simulink model "sampleModel1903"  (R2023a)
settings: Solver=VariableStepAuto  StartTime=0.0  StopTime=10.0  RelTol=1e-3
libraries: hdlsllib x2, simulink x1
settings Model: Creator=user1  LastModifiedBy=user1

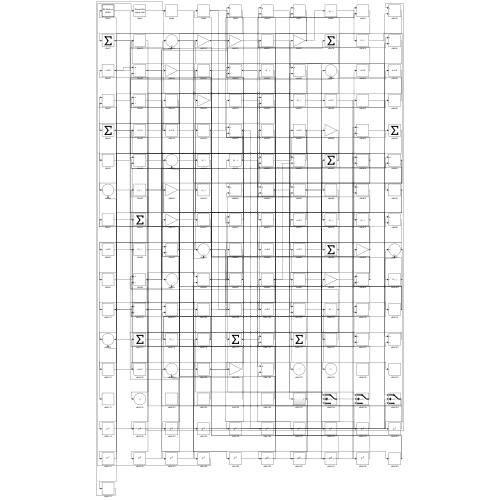
[thumbnail: Simulink's stored preview of the top-level diagram]
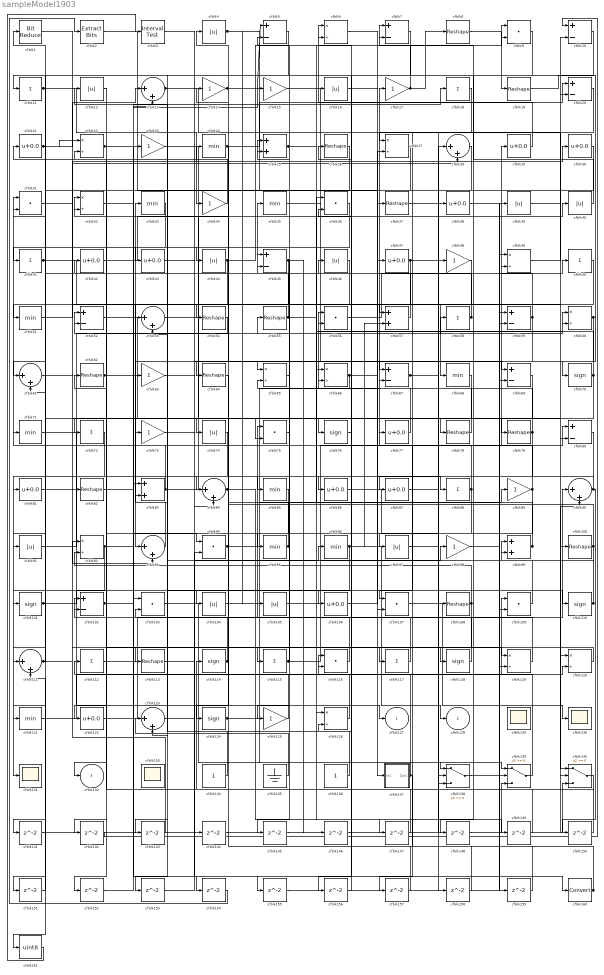
== system sampleModel1903 ==
  cfblk1 : hdlsllib/Logic and Bit Operations/Bit Reduce  mode=AND
  cfblk{5,7,10,20,45,52,59,67,69,80,102} (11 alike) : Sum  Inputs=+-
  cfblk{8,19,26,37,54..55,62,64,78..79,82,100,108,113} (14 alike) : Reshape
  cfblk{70,76,101,110,114,118,124} (7 alike) : Signum
  cfblk{9,31,36,56,75,94,103,107,109,116} (10 alike) : DotProduct  OutDataTypeStr=Inherit: Inherit via internal rule
  cfblk{4,12,16,39..40,44,46,74,91,97,104..105} (12 alike) : Abs  SaturateOnIntegerOverflow=off
  cfblk{21,29..30,38,42..43,47,77,81,86..87,106,122} (13 alike) : Bias  Bias=0.0  SaturateOnIntegerOverflow=off
  cfblk{11,18,41,50,58,72,88,112,115,117} (10 alike) : Sum  Inputs=+
  cfblk{13,28,53,61,84,90,93,111,123} (9 alike) : Sum  Inputs=|++
  cfblk{6,22,27,32,49,60,65..66,92,119..120,126} (12 alike) : Product  Inputs=*/  RndMeth=Zero  SaturateOnIntegerOverflow=on
  cfblk{24,33,35,51,68,71,85,95..96,121} (10 alike) : MinMax
  cfblk{14..15,17,23,34,48,63,73,89,98,125} (11 alike) : Gain
  cfblk{129..131,133} (4 alike) : Scope
      cfblk129 settings: Floating=on
      cfblk133 settings: Floating=on
  cfblk134 : Constant  SampleTime=-1
  cfblk135 : Ground
  cfblk136 : Constant  SampleTime=-1
  cfblk137 : Subsystem
      settings: LibrarySourceBlock=|
      | hdlsllib/Ports &
      | Subsystems/Subsystem
  cfblk138 : Switch  SaturateOnIntegerOverflow=off  InputSameDT=off
  cfblk139 : Switch  SaturateOnIntegerOverflow=off  InputSameDT=off
  cfblk140 : Switch  SaturateOnIntegerOverflow=off  InputSameDT=off
  cfblk{141..159} (19 alike) : Delay  SampleTime=1
  cfblk160 : DataTypeConversion  SaturateOnIntegerOverflow=off  RndMeth=Floor
  cfblk161 : DataTypeConversion  OutDataTypeStr=uint8  SaturateOnIntegerOverflow=off  RndMeth=Floor
  cfblk2 : simulink/Logic and Bit Operations/Extract Bits  bitsToExtract=Upper half  numBits=8  bitIdxRange=[0 7]  outScalingMode=Preserve fixed-point scaling
      settings: LibrarySourceBlock=|
      | hdlsllib/Logic and Bit
      | Operations/Extract Bits
  cfblk{25,57,83,99} (4 alike) : Sum
  cfblk3 : hdlsllib/Logic and Bit Operations/Interval Test  IntervalClosedRight=on  uplimit=0.5  IntervalClosedLeft=on  lowlimit=-0.5  OutDataTypeStr=boolean
  cfblk127 : Outport  VectorParamsAs1DForOutWhenUnconnected=off
  cfblk128 : Outport  Port=2  VectorParamsAs1DForOutWhenUnconnected=off
  cfblk132 : Outport  Port=3  VectorParamsAs1DForOutWhenUnconnected=off
  wires:
  cfblk103/1 -> cfblk139/1
  cfblk89/1 -> cfblk17/1, cfblk62/1, cfblk95/1
  cfblk35/1 -> cfblk67/1
  cfblk23/1 -> cfblk76/1
  cfblk57/1 -> cfblk35/1
  cfblk24/1 -> cfblk20/1, cfblk64/1
  cfblk118/1 -> cfblk31/1
  cfblk140/1 -> cfblk114/1
  cfblk4/1 -> cfblk137/1(In1), cfblk105/1
  cfblk25/1 -> cfblk9/2, cfblk147/1
  cfblk21/1 -> cfblk22/1, cfblk13/1
  cfblk56/1 -> cfblk50/1
  cfblk14/1 -> cfblk5/1, cfblk38/1
  cfblk122/1 -> cfblk90/1
  cfblk94/1 -> cfblk89/1, cfblk47/1
  cfblk20/1 -> cfblk27/1
  cfblk95/1 -> cfblk52/1, cfblk125/1
  cfblk124/1 -> cfblk67/2, cfblk138/2
  cfblk135/1 -> cfblk123/1
  cfblk71/1 -> cfblk127/1
  cfblk19/1 -> cfblk70/1
  cfblk111/1 -> cfblk21/1, cfblk117/1
  cfblk11/1 -> cfblk34/1, cfblk75/2
  cfblk100/1 -> cfblk24/1, cfblk99/2
  cfblk115/1 -> cfblk98/1, cfblk25/2
  cfblk72/1 -> cfblk131/1
  cfblk91/1 -> cfblk60/1
  cfblk105/1 -> cfblk29/1
  cfblk49/1 -> cfblk20/2
  cfblk107/1 -> cfblk130/1
  cfblk7/1 -> cfblk86/1
  cfblk93/1 -> cfblk33/1
  cfblk13/1 -> cfblk100/1, cfblk155/1
  cfblk96/1 -> cfblk128/1, cfblk57/2, cfblk113/1, cfblk46/1
  cfblk97/1 -> cfblk48/1
  cfblk77/1 -> cfblk56/1
  cfblk88/1 -> cfblk97/1, cfblk42/1
  cfblk36/1 -> cfblk41/1
  cfblk84/1 -> cfblk107/2, cfblk149/1
  cfblk3/1 -> cfblk160/1
  cfblk42/1 -> cfblk40/1
  cfblk83/1 -> cfblk10/2, cfblk61/2
  cfblk54/1 -> cfblk52/2
  cfblk39/1 -> cfblk140/1
  cfblk101/1 -> cfblk104/1, cfblk118/1
  cfblk2/1 -> cfblk126/1
  cfblk10/1 -> cfblk111/1
  cfblk102/1 -> cfblk23/1, cfblk58/1
  cfblk106/1 -> cfblk27/2
  cfblk6/1 -> cfblk37/1
  cfblk86/1 -> cfblk108/1
  cfblk112/1 -> cfblk39/1
  cfblk47/1 -> cfblk93/1, cfblk61/1, cfblk80/2
  cfblk16/1 -> cfblk88/1
  cfblk92/1 -> cfblk18/1, cfblk15/1, cfblk151/1
  cfblk109/1 -> cfblk12/1
  cfblk46/1 -> cfblk51/1
  cfblk125/1 -> cfblk73/1
  cfblk64/1 -> cfblk124/1
  cfblk59/1 -> cfblk57/1, cfblk69/2, cfblk65/1, cfblk49/2
  cfblk28/1 -> cfblk44/1
  cfblk139/1 -> cfblk112/1
  cfblk22/1 -> cfblk94/1, cfblk13/2
  cfblk119/1 -> cfblk75/1
  cfblk70/1 -> cfblk79/1, cfblk121/1, cfblk26/1
  cfblk90/1 -> cfblk81/1, cfblk150/1
  cfblk29/1 -> cfblk6/1
  cfblk52/1 -> cfblk78/1
  cfblk8/1 -> cfblk19/1
  cfblk51/1 -> cfblk30/1
  cfblk15/1 -> cfblk120/1
  cfblk18/1 -> cfblk87/1
  cfblk1/1 -> cfblk53/1
  cfblk43/1 -> cfblk69/1
  cfblk121/1 -> cfblk109/1
  cfblk34/1 -> cfblk1/1
  cfblk81/1 -> cfblk110/1
  cfblk79/1 -> cfblk106/1, cfblk5/2
  cfblk87/1 -> cfblk80/1
  cfblk62/1 -> cfblk74/1, cfblk55/1
  cfblk123/1 -> cfblk96/1
  cfblk17/1 -> cfblk7/1, cfblk8/1, cfblk11/1
  cfblk136/1 -> cfblk71/1
  cfblk53/1 -> cfblk109/2
  cfblk113/1 -> cfblk120/2
  cfblk138/1 -> cfblk49/1
  cfblk44/1 -> cfblk122/1, cfblk9/1
  cfblk58/1 -> cfblk54/1, cfblk45/2
  cfblk40/1 -> cfblk7/2
  cfblk50/1 -> cfblk68/1
  cfblk67/1 -> cfblk119/1, cfblk119/2
  cfblk80/1 -> cfblk101/1
  cfblk65/1 -> cfblk85/1
  cfblk48/1 -> cfblk107/1
  cfblk41/1 -> cfblk66/1, cfblk93/2
  cfblk12/1 -> cfblk72/1
  cfblk66/1 -> cfblk138/1, cfblk65/2
  cfblk98/1 -> cfblk59/1
  cfblk114/1 -> cfblk83/2, cfblk102/1
  cfblk32/1 -> cfblk59/2
  cfblk30/1 -> cfblk43/1
  cfblk60/1 -> cfblk63/1, cfblk138/3
  cfblk78/1 -> cfblk16/1
  cfblk69/1 -> cfblk84/1
  cfblk104/1 -> cfblk36/1
  cfblk73/1 -> cfblk84/2
  cfblk134/1 -> cfblk32/1
  cfblk137/1(Out1) -> cfblk102/2, cfblk157/1
  cfblk120/1 -> cfblk115/1
  cfblk99/1 -> cfblk32/2, cfblk66/2
  cfblk45/1 -> cfblk91/1, cfblk145/1, cfblk146/1
  cfblk75/1 -> cfblk25/1
  cfblk108/1 -> cfblk132/1, cfblk92/2
  cfblk110/1 -> cfblk45/1, cfblk99/1, cfblk53/2
  cfblk31/1 -> cfblk28/2
  cfblk116/1 -> cfblk103/2
  cfblk5/1 -> cfblk123/2
  cfblk126/1 -> cfblk116/1
  cfblk61/1 -> cfblk82/1
  cfblk117/1 -> cfblk36/2
  cfblk55/1 -> cfblk31/2, cfblk60/2
  cfblk27/1 -> cfblk141/1
  cfblk141/1 -> cfblk140/3
  cfblk85/1 -> cfblk142/1
  cfblk142/1 -> cfblk10/1
  cfblk68/1 -> cfblk143/1
  cfblk143/1 -> cfblk92/1
  cfblk63/1 -> cfblk144/1
  cfblk144/1 -> cfblk28/1
  cfblk145/1 -> cfblk90/2
  cfblk146/1 -> cfblk139/3
  cfblk147/1 -> cfblk103/1
  cfblk9/1 -> cfblk148/1
  cfblk148/1 -> cfblk140/2
  cfblk149/1 -> cfblk22/2
  cfblk150/1 -> cfblk116/2
  cfblk151/1 -> cfblk111/2
  cfblk26/1 -> cfblk152/1
  cfblk152/1 -> cfblk83/1
  cfblk74/1 -> cfblk153/1
  cfblk153/1 -> cfblk94/2
  cfblk82/1 -> cfblk154/1
  cfblk154/1 -> cfblk2/1
  cfblk155/1 -> cfblk139/2
  cfblk76/1 -> cfblk156/1
  cfblk156/1 -> cfblk126/2
  cfblk157/1 -> cfblk4/1
  cfblk37/1 -> cfblk158/1
  cfblk158/1 -> cfblk6/2
  cfblk38/1 -> cfblk159/1
  cfblk159/1 -> cfblk14/1
  cfblk160/1 -> cfblk56/2, cfblk77/1
  cfblk33/1 -> cfblk161/1
  cfblk161/1 -> cfblk3/1

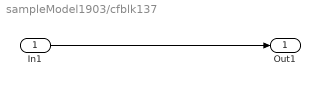
== system sampleModel1903/cfblk137 ==
  In1 : Inport
  Out1 : Outport
  wires:
  In1/1 -> Out1/1
